simulink model "Two_Level_SVM_No_PV_No_Control_Average_Benchmark_v2"  (R2022b)
settings: Solver=FixedStepAuto  StartTime=0.0  StopTime=5  FixedStep=1e-7  RelTol=1e-3
model workspace (MAT data in the model file):
  Phase_Shift = Simulink.Parameter
  Phase_Shift.Value = 0.1974
  Phase_Shift.DataType = 'auto'
  Phase_Shift.Complexity = 'real'
  Phase_Shift.Dimensions = [1 1]
  Vrms_p = Simulink.Parameter
  Vrms_p.Value = 285.7229
  Vrms_p.DataType = 'auto'
  Vrms_p.Complexity = 'real'
  Vrms_p.Dimensions = [1 1]
libraries: slpidlib x5, spsThreePhaseSeriesRLCBranchLib x4, spsThreePhaseVIMeasurementLib x4, spsControlledCurrentSourceLib x3, spsControlledVoltageSourceLib x3, spsGroundLib x2, spsabctodq0Lib x2, spsdq0toabcLib x1, spsDCVoltageSourceLib x1, spsThreePhaseProgrammableVoltageSourceLib x1, eeGeneralControl x1, spsabctoAlphaBetaZeroLib x1
settings Model: Creator=Jacob  LastModifiedBy=buckb
settings ModelReferenceCC: EnableRefExpFcnMdlSchedulingChecks=on

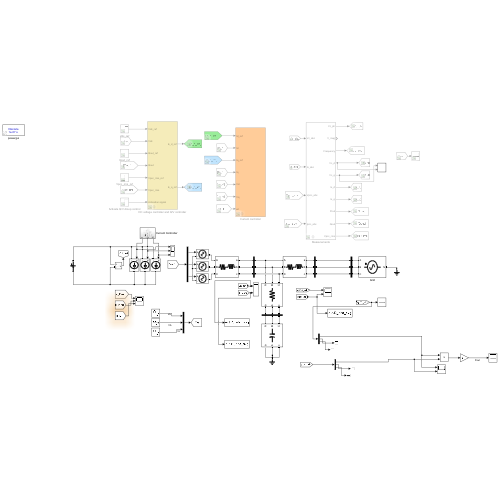
[thumbnail: Simulink's stored preview of the top-level diagram]
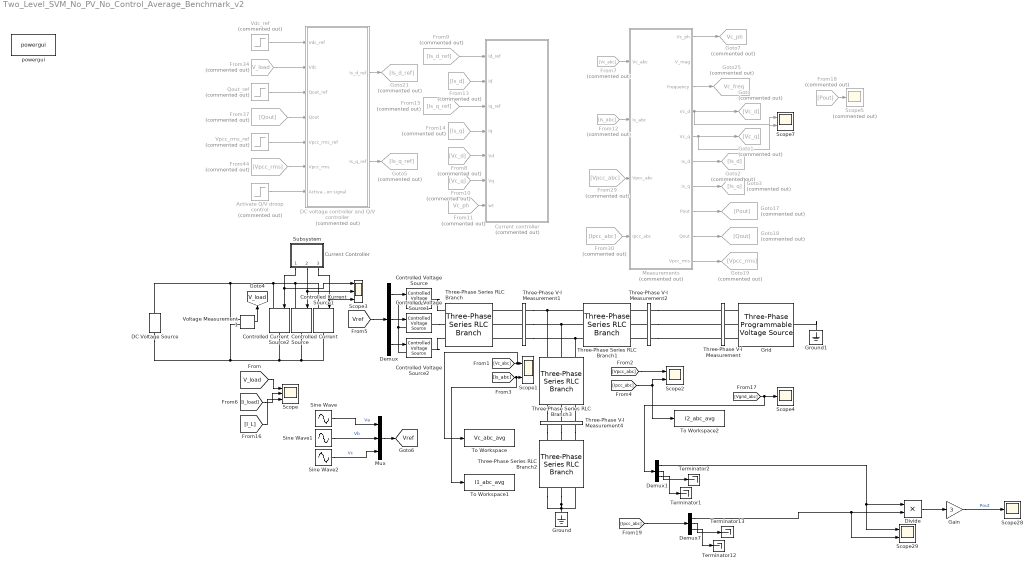
== system Two_Level_SVM_No_PV_No_Control_Average_Benchmark_v2 ==
  note: Current Controller
  Activate Q/V droop control : Step  Commented=on  Time=3  After=0  SampleTime=0
  Controlled Current Source : spsControlledCurrentSourceLib/Controlled Current Source  Initialize=on  Source_Type=AC  Amplitude=0  Phase=0  Frequency=0  Measurements=None
  Controlled Current Source1 : spsControlledCurrentSourceLib/Controlled Current Source  Initialize=on  Source_Type=AC  Amplitude=0  Phase=0  Frequency=0  Measurements=None
  Controlled Current Source2 : spsControlledCurrentSourceLib/Controlled Current Source  Initialize=on  Source_Type=AC  Amplitude=0  Phase=0  Frequency=0  Measurements=None
  Controlled Voltage Source : spsControlledVoltageSourceLib/Controlled Voltage Source  Initialize=on  Source_Type=AC  Amplitude=0  Phase=0  Frequency=0  Measurements=None
  Controlled Voltage Source1 : spsControlledVoltageSourceLib/Controlled Voltage Source  Initialize=on  Source_Type=AC  Amplitude=0  Phase=0  Frequency=0  Measurements=None
  Controlled Voltage Source2 : spsControlledVoltageSourceLib/Controlled Voltage Source  Initialize=on  Source_Type=AC  Amplitude=0  Phase=0  Frequency=0  Measurements=None
  Current controller : Subsystem  Commented=on  mask{Kp_current_loop=0.59, Ki_current_loop=30, L1=3e-03}
      mask prompts: Kp_current_loop "Proportional parameter of current loop"; Ki_current_loop "Integral parameter of current loop"; L1 "Inverter-side inductor value [H]"
      mask TypeOptions Kp_current_loop: Discrete PID Controller/P | Discrete PID Controller1/P
      mask TypeOptions Ki_current_loop: Discrete PID Controller/I | Discrete PID Controller1/I
      mask TypeOptions L1: L/Gain | L1/Gain
  DC Voltage Source : spsDCVoltageSourceLib/DC Voltage Source  Amplitude=1000  Measurements=None
  DC voltage controller and Q/V controller : Subsystem  Commented=on  mask(DC voltage controller and Q/V controller){Kp_vdc_control=0.05, Ki_vdc_control=10, Kp_QV_control=1e-3, Ki_QV_control=1e-2, Dq=4.1667e+03}
      mask prompts: Kp_vdc_control "Proportional parameter of DC voltage controller"; Ki_vdc_control "Integral parameter of DC voltage controller"; Kp_QV_control "Proportional parameter of Q/V controller"; Ki_QV_control "Integral parameter of Q/V controller"; Dq "Q/V droop constant [Var/V]"
      mask TypeOptions Kp_vdc_control: Discrete PID Controller/P
      mask TypeOptions Ki_vdc_control: Discrete PID Controller/I
      mask TypeOptions Kp_QV_control: Discrete PID Controller3/P
      mask TypeOptions Ki_QV_control: Discrete PID Controller3/I
      mask TypeOptions Dq: Dq/Gain
      mask DialogControl ParameterGroupVar1 Prompt: DC voltage controller
      mask DialogControl ParameterGroupVar2 Prompt: Q/V controller
  Demux : Demux  Outputs=3
  Demux1 : Demux  Outputs=3
  Demux7 : Demux  Outputs=3
  Divide : Product  Inputs=**
  From10 : From  Commented=on  GotoTag=Vc_q
  From11 : From  Commented=on  GotoTag=Vc_ph  TagVisibility=global
  From12 : From  Commented=on  GotoTag=Is_abc  TagVisibility=global
  From13 : From  Commented=on  GotoTag=Is_d
  From14 : From  Commented=on  GotoTag=Is_q
  From15 : From  Commented=on  GotoTag=Is_q_ref
  From18 : From  Commented=on  GotoTag=Pout
  From29 : From  Commented=on  GotoTag=Vpcc_abc  TagVisibility=global
  From30 : From  Commented=on  GotoTag=Ipcc_abc  TagVisibility=global
  From34 : From  Commented=on  GotoTag=V_load  TagVisibility=global
  From37 : From  Commented=on  GotoTag=Qout
  From44 : From  Commented=on  GotoTag=Vpcc_rms
  From7 : From  Commented=on  GotoTag=Vc_abc  TagVisibility=global
  From8 : From  Commented=on  GotoTag=Vc_d
  From9 : From  Commented=on  GotoTag=Is_d_ref
  Gain : Gain  Gain=3
  Goto : Goto  Commented=on  GotoTag=Vc_d
  Goto1 : Goto  Commented=on  GotoTag=Vc_q
  Goto17 : Goto  Commented=on  GotoTag=Pout
  Goto18 : Goto  Commented=on  GotoTag=Qout
  Goto19 : Goto  Commented=on  GotoTag=Vpcc_rms
  Goto2 : Goto  Commented=on  GotoTag=Is_d
  Goto21 : Goto  Commented=on  GotoTag=Is_d_ref
  Goto25 : Goto  Commented=on  GotoTag=Vc_freq  TagVisibility=global
  Goto3 : Goto  Commented=on  GotoTag=Is_q
  Goto5 : Goto  Commented=on  GotoTag=Is_q_ref
  Goto7 : Goto  Commented=on  GotoTag=Vc_ph  TagVisibility=global
  Grid : spsThreePhaseProgrammableVoltageSourceLib/Three-Phase Programmable Voltage Source  PositiveSequence="[480  0 60]"  VariationEntity=None  VariationType=Table of time-amplitude pairs  VariationTypeAlt=Step  VariationStep=-0.1  VariationRate=10  VariationMagnitude=0.3  VariationFrequency=2  VariationTiming=[5.5 6.5]  VariationPhaseA=off  Amplitudes=[1 0.96 1.02]  TimeValues=[0 7 8.5]  HarmonicGeneration=off  HarmonicA=[3 0.2 -25 0]  HarmonicB=[2 0.15 35 2]  Timing="[0.05  3]"  BusType=swing  Pref=0  Qref=0  Qmin=-inf  Qmax=inf
  Ground : spsGroundLib/Ground  LConnTagsString=a
  Ground1 : spsGroundLib/Ground  LConnTagsString=a
  Measurements : Subsystem  Commented=on  mask{Kp_PLL=100, Ki_PLL=1e5}
      mask prompts: Kp_PLL "Proportional parameter of PLL"; Ki_PLL "Integral parameter of PLL"
      mask TypeOptions Kp_PLL: Phase Locked Loop (PLL)/Discrete PID Controller/P
      mask TypeOptions Ki_PLL: Phase Locked Loop (PLL)/Discrete PID Controller/I
  Mux : Mux  Inputs=3
  Qout_ref : Step  Commented=on  Time=0  After=0  SampleTime=0
  Scope : Scope  NumInputPorts=3
  Scope{1..2,7,29} (4 alike) : Scope  NumInputPorts=2
  Scope28 : Scope
  Scope3 : Scope  NumInputPorts=3
  Scope4 : Scope
  Scope5 : Scope  Commented=on
  Sine Wave : Sin  Amplitude=Vrms_p*sqrt(2)  Frequency=2*pi*60  Phase=Phase_Shift  SampleTime=0
  Sine Wave1 : Sin  Amplitude=Vrms_p*sqrt(2)  Frequency=2*pi*60  Phase=4*pi/3+Phase_Shift  SampleTime=0
  Sine Wave2 : Sin  Amplitude=Vrms_p*sqrt(2)  Frequency=2*pi*60  Phase=2*pi/3+Phase_Shift  SampleTime=0
  Subsystem : Subsystem
  Terminator{1..2,12..13} (4 alike) : Terminator
  Three-Phase Series RLC Branch : spsThreePhaseSeriesRLCBranchLib/Three-Phase Series RLC Branch  LConnTagsString=A|B|C  RConnTagsString=A|B|C  BranchType=RL  Resistance=0.03  Inductance=3e-04  Capacitance=1e-6  Measurements=None
  Three-Phase Series RLC Branch1 : spsThreePhaseSeriesRLCBranchLib/Three-Phase Series RLC Branch  LConnTagsString=A|B|C  RConnTagsString=A|B|C  BranchType=RL  Resistance=0.0053  Inductance=9.3183e-04  Capacitance=1e-6  Measurements=None
  Three-Phase Series RLC Branch2 : spsThreePhaseSeriesRLCBranchLib/Three-Phase Series RLC Branch  LConnTagsString=A|B|C  RConnTagsString=A|B|C  BranchType=C  Resistance=1  Inductance=1e-3  Capacitance=9.7860e-5  Measurements=None
  Three-Phase Series RLC Branch3 : spsThreePhaseSeriesRLCBranchLib/Three-Phase Series RLC Branch  LConnTagsString=A|B|C  RConnTagsString=A|B|C  BranchType=R  Resistance=1  Inductance=1e-3  Capacitance=9.7860e-5  Measurements=None
  Three-Phase V-I Measurement : spsThreePhaseVIMeasurementLib/Three-Phase V-I Measurement  VoltageMeasurement=phase-to-ground  SetLabelV=on  LabelV=Vgrid_abc  Vpu=off  VpuLL=off  CurrentMeasurement=yes  SetLabelI=on  LabelI=Igrid_abc  Ipu=off  Pbase=100e6  Vbase=500e3  OutputType=Complex  PhasorSimulation=off  PSBequivalent=0
  Three-Phase V-I Measurement1 : spsThreePhaseVIMeasurementLib/Three-Phase V-I Measurement  VoltageMeasurement=phase-to-ground  SetLabelV=on  LabelV=Vrc_abc  Vpu=off  VpuLL=off  CurrentMeasurement=yes  SetLabelI=on  LabelI=Is_abc  Ipu=off  Pbase=100e6  Vbase=500e3  OutputType=Complex  PhasorSimulation=off  PSBequivalent=0
  Three-Phase V-I Measurement2 : spsThreePhaseVIMeasurementLib/Three-Phase V-I Measurement  VoltageMeasurement=phase-to-ground  SetLabelV=on  LabelV=Vpcc_abc  Vpu=off  VpuLL=off  CurrentMeasurement=yes  SetLabelI=on  LabelI=Ipcc_abc  Ipu=off  Pbase=100e6  Vbase=500e3  OutputType=Complex  PhasorSimulation=off  PSBequivalent=0
  Three-Phase V-I Measurement4 : spsThreePhaseVIMeasurementLib/Three-Phase V-I Measurement  VoltageMeasurement=phase-to-ground  SetLabelV=on  LabelV=Vc_abc  Vpu=off  VpuLL=off  CurrentMeasurement=yes  SetLabelI=on  LabelI=Ic_abc  Ipu=off  Pbase=100e6  Vbase=500e3  OutputType=Complex  PhasorSimulation=off  PSBequivalent=0
  To Workspace : ToWorkspace  VariableName=Vc_abc_avg  SaveFormat=Timeseries  SampleTime=-1
  To Workspace1 : ToWorkspace  VariableName=I1_abc_avg  SaveFormat=Timeseries  SampleTime=-1
  To Workspace2 : ToWorkspace  VariableName=I2_abc_avg  SaveFormat=Timeseries  SampleTime=-1
  Vdc_ref : Step  Commented=on  Time=0.5  Before=1000  After=1000  SampleTime=0
  Voltage Measurement1 : spsVoltageMeasurementLib/Voltage Measurement  PhasorSimulation=off  OutputType=Complex  PSBequivalent=0
  Vpcc_rms_ref : Step  Commented=on  Time=0.5  Before=480  After=480  SampleTime=0
  powergui : spspowerguiLib/powergui  Priority=1  SimulationMode=Discrete  SampleTime=1e-7  frequency=60  Iterations=50  frequencyindice=0  Pbase=100e6  ErrMax=1e-4  UnitsV=kV  UnitsW=MW  buscounter=0  FunctionMessages=off  echomessages=off  EnableUseOfTLC=off  CurrentSourceSwitches=off  DisableSnubberDevices=off  DisableRonSwitches=off  DisableVfSwitches=off  DisplayEquations=off  AutomaticDiscreteSolvers=off  SolverType=Tustin/Backward Euler (TBE)  Interpol=off  ExternalGateDelay=off  methode=off  Ts=100  x0status=blocks  SPID=on  SwTol=0  HookPort=off  NonlinearTolerance=1e-4  nMaxIteration=100  ContinueOnMaxIteration=off  RestoreLinks=warning  ResistiveCurrentMeasurement=off  Frange=[0:2:500]  Ylog=off  Xlog=on  ShowGrid=off  save=off  variable=ZData  structure=0  ZoomFFT=off  StartTime=0.0  cycles=1  DisplayStyle=1  fundamental=60  FreqAxis=off  MaxFrequency=1000  frequencyindicesteady=1  RmsSteady=1  display=off
  tag scope: V_load=global, Vref=global
  wires:
  Voltage Measurement1/1 -> [V_load]
  [V_load] -> Scope/1
  [Vpcc_abc] -> Scope2/1
  [Ipcc_abc] -> To Workspace2/1, Scope2/2
  Subsystem/1(Out1) -> Controlled Current Source2/1, Scope3/1
  Subsystem/2(Out2) -> Controlled Current Source/1, Scope3/2
  Subsystem/3(Out3) -> Controlled Current Source1/1, Scope3/3
  Demux/1 -> Controlled Voltage Source/1
  Demux/2 -> Controlled Voltage Source1/1
  Demux/3 -> Controlled Voltage Source2/1
  From8/1 -> Current controller/5(Vd)
  From10/1 -> Current controller/6(Vq)
  From11/1 -> Current controller/7(wt)
  From14/1 -> Current controller/4(Iq)
  From13/1 -> Current controller/2(Id)
  From7/1 -> Measurements/1(Vc_abc)
  From12/1 -> Measurements/2(Is_abc)
  Measurements/4(Vc_d) -> Scope7/1, Goto/1
  Measurements/5(Vc_q) -> Scope7/2, Goto1/1
  Measurements/6(Is_d) -> Goto2/1
  Measurements/7(Is_q) -> Goto3/1
  Qout_ref/1 -> DC voltage controller and Q/V controller/3(Qout_ref)
  From44/1 -> DC voltage controller and Q/V controller/6(Vpcc_rms)
  DC voltage controller and Q/V controller/2(Is_q_ref) -> Goto5/1
  Activate Q/V droop control/1 -> DC voltage controller and Q/V controller/7(Activation signal)
  Vpcc_rms_ref/1 -> DC voltage controller and Q/V controller/5(Vpcc_rms_ref)
  From37/1 -> DC voltage controller and Q/V controller/4(Qout)
  DC voltage controller and Q/V controller/1(Is_d_ref) -> Goto21/1
  Vdc_ref/1 -> DC voltage controller and Q/V controller/1(Vdc_ref)
  From29/1 -> Measurements/3(Vpcc_abc)
  From30/1 -> Measurements/4(Ipcc_abc)
  Measurements/8(Pout) -> Goto17/1
  Measurements/9(Qout) -> Goto18/1
  Measurements/10(Vpcc_rms) -> Goto19/1
  Measurements/3(Frequency) -> Goto25/1
  From15/1 -> Current controller/3(Iq_ref)
  From9/1 -> Current controller/1(Id_ref)
  Measurements/1(Vc_ph) -> Goto7/1
  From18/1 -> Scope5/1
  [I_L] -> Scope/3
  [I_load] -> Scope/2
  From34/1 -> DC voltage controller and Q/V controller/2(Vdc)
  [Is_abc] -> To Workspace1/1, Scope1/2
  [Vc_abc] -> To Workspace/1, Scope1/1
  Sine Wave1/1 -> Mux/2  "Vb"
  Sine Wave/1 -> Mux/1  "Va"
  Sine Wave2/1 -> Mux/3  "Vc"
  Mux/1 -> [Vref]
  [Vref] -> Demux/1
  Demux7/2 -> Terminator13/1
  Demux7/1 -> Scope29/2, Divide/2
  Demux1/1 -> Scope29/1, Divide/1
  Demux7/3 -> Terminator12/1
  [Ipcc_abc] -> Demux7/1
  Gain/1 -> Scope28/1  "Pout"
  Divide/1 -> Gain/1
  Demux1/3 -> Terminator1/1
  Demux1/2 -> Terminator2/1
  [Vgrid_abc] -> Demux1/1, Scope4/1
  connections:
  DC Voltage Source/RConn1 -- Voltage Measurement1/LConn1 -- Controlled Current Source2/LConn1 -- Controlled Current Source1/LConn1 -- Controlled Current Source/LConn1
  Three-Phase V-I Measurement1/RConn3 -- Three-Phase Series RLC Branch3/LConn3 -- Three-Phase Series RLC Branch1/LConn3
  Three-Phase V-I Measurement1/RConn1 -- Three-Phase Series RLC Branch3/LConn1 -- Three-Phase Series RLC Branch1/LConn1
  Three-Phase V-I Measurement1/RConn2 -- Three-Phase Series RLC Branch3/LConn2 -- Three-Phase Series RLC Branch1/LConn2
  Three-Phase V-I Measurement1/LConn3 -- Three-Phase Series RLC Branch/RConn3
  Three-Phase V-I Measurement2/RConn3 -- Three-Phase V-I Measurement/LConn3
  Three-Phase V-I Measurement2/RConn1 -- Three-Phase V-I Measurement/LConn1
  Grid/RConn1 -- Three-Phase V-I Measurement/RConn1
  Grid/RConn2 -- Three-Phase V-I Measurement/RConn2
  Ground1/LConn1 -- Grid/LConn1
  Three-Phase V-I Measurement1/LConn1 -- Three-Phase Series RLC Branch/RConn1
  Grid/RConn3 -- Three-Phase V-I Measurement/RConn3
  Three-Phase V-I Measurement1/LConn2 -- Three-Phase Series RLC Branch/RConn2
  Three-Phase V-I Measurement2/RConn2 -- Three-Phase V-I Measurement/LConn2
  Controlled Voltage Source/LConn1 -- Controlled Voltage Source2/LConn1 -- Controlled Voltage Source1/LConn1
  Controlled Voltage Source/RConn1 -- Three-Phase Series RLC Branch/LConn1
  Controlled Voltage Source1/RConn1 -- Three-Phase Series RLC Branch/LConn2
  Controlled Voltage Source2/RConn1 -- Three-Phase Series RLC Branch/LConn3
  Three-Phase V-I Measurement2/LConn1 -- Three-Phase Series RLC Branch1/RConn1
  Three-Phase V-I Measurement2/LConn2 -- Three-Phase Series RLC Branch1/RConn2
  Three-Phase V-I Measurement2/LConn3 -- Three-Phase Series RLC Branch1/RConn3
  Controlled Current Source/RConn1 -- Controlled Current Source1/RConn1 -- Controlled Current Source2/RConn1 -- DC Voltage Source/LConn1 -- Voltage Measurement1/LConn2
  Ground/LConn1 -- Three-Phase Series RLC Branch2/RConn1 -- Three-Phase Series RLC Branch2/RConn3 -- Three-Phase Series RLC Branch2/RConn2
  Three-Phase V-I Measurement4/LConn3 -- Three-Phase Series RLC Branch3/RConn3
  Three-Phase Series RLC Branch3/RConn2 -- Three-Phase V-I Measurement4/LConn2
  Three-Phase Series RLC Branch3/RConn1 -- Three-Phase V-I Measurement4/LConn1
  Three-Phase V-I Measurement4/RConn1 -- Three-Phase Series RLC Branch2/LConn1
  Three-Phase V-I Measurement4/RConn2 -- Three-Phase Series RLC Branch2/LConn2
  Three-Phase V-I Measurement4/RConn3 -- Three-Phase Series RLC Branch2/LConn3

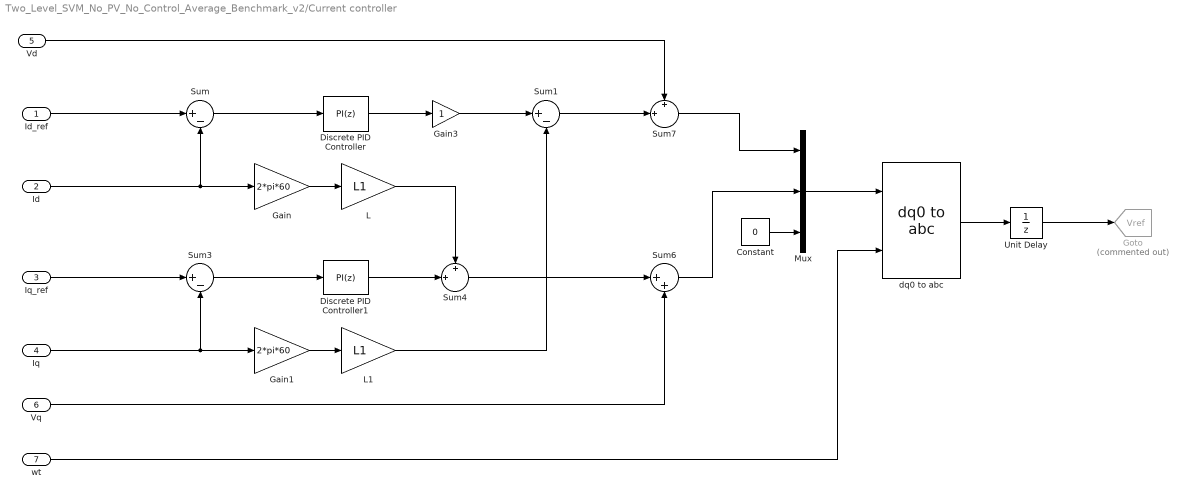
== system Two_Level_SVM_No_PV_No_Control_Average_Benchmark_v2/Current controller ==
  Id_ref : Inport
  Id : Inport  Port=2
  Iq_ref : Inport  Port=3
  Iq : Inport  Port=4
  Vd : Inport  Port=5
  Vq : Inport  Port=6
  wt : Inport  Port=7
  Constant : Constant  Value=0
  Discrete PID Controller : slpidlib/PID Controller  Controller=PI  Form=Parallel  TimeDomain=Discrete-time  UseExternalTs=off  SampleTime=-1  IntegratorMethod=Forward Euler  FilterMethod=Forward Euler  ControllerParametersSource=internal  P=Kp_current_loop  I=Ki_current_loop  UseKiTs=off  D=0  N=100  UseFilter=on  TunerSelectOption=Transfer Function Based (PID Tuner App)  InitialConditionSource=internal  InitialConditionForIntegrator=0  InitialConditionForFilter=0  DifferentiatorICPrevScaledInput=0  ExternalReset=none  TrackingMode=off  Kt=1  LimitOutput=off  SatLimitsSource=internal  UpperSaturationLimit=inf  LowerSaturationLimit=-inf  LinearizeAsGain=off  AntiWindupMode=none  Kb=1  LimitIntegrator=off  UpperIntegratorSaturationLimit=inf  LowerIntegratorSaturationLimit=-inf  POutMin=[]  POutMax=[]  IOutMin=[]  IOutMax=[]  DOutMin=[]  DOutMax=[]  NOutMin=[]  NOutMax=[]  SumOutMin=[]  SumOutMax=[]  SaturationOutMin=[]  SaturationOutMax=[]  PParamMin=[]  PParamMax=[]  IParamMin=[]  IParamMax=[]  DParamMin=[]  DParamMax=[]  NParamMin=[]  NParamMax=[]  KbParamMin=[]  KbParamMax=[]  KtParamMin=[]  KtParamMax=[]  KbOutMin=[]  KbOutMax=[]  KtOutMin=[]  KtOutMax=[]  IntegratorOutMin=[]  IntegratorOutMax=[]  FilterOutMin=[]  FilterOutMax=[]  SumI1OutMin=[]  SumI1OutMax=[]  SumI2OutMin=[]  SumI2OutMax=[]  SumI3OutMin=[]  SumI3OutMax=[]  SumI4OutMin=[]  SumI4OutMax=[]  SumDOutMin=[]  SumDOutMax=[]  DifferentiatorOutMin=[]  DifferentiatorOutMax=[]  FilterDiffOutCoefMin=[]  FilterDiffOutCoefMax=[]  ReciprocalOutMin=[]  ReciprocalOutMax=[]  SumDenOutMin=[]  SumDenOutMax=[]  SumNumOutMin=[]  SumNumOutMax=[]  DivideOutMin=[]  DivideOutMax=[]  UdiffTsProdOutMin=[]  UdiffTsProdOutMax=[]  NTsProdOutMin=[]  NTsProdOutMax=[]  UintegralTsProdOutMin=[]  UintegralTsProdOutMax=[]  UngainTsProdOutMin=[]  UngainTsProdOutMax=[]  ClampingZeroOutDataTypeStr=Inherit: Inherit via back propagation  ClampingZeroOutMin=[]  ClampingZeroOutMax=[]  FilterDenConstantOutDataTypeStr=Inherit: Inherit via back propagation  FilterDenConstantOutMin=[]  FilterDenConstantOutMax=[]  PCopyOutDataTypeStr=Inherit: Inherit via back propagation  PCopyOutMin=[]  PCopyOutMax=[]  NCopyOutDataTypeStr=Inherit: Inherit via back propagation  NCopyOutMin=[]  NCopyOutMax=[]  IntegratorContinuousStateAttributes=''  IntegratorStateMustResolveToSignalObject=off  IntegratorRTWStateStorageClass=Auto  FilterContinuousStateAttributes=''  FilterStateMustResolveToSignalObject=off  FilterRTWStateStorageClass=Auto  ParallelPVariant=InternalParameters  IdealPVariant=Disabled  IVariant=InternalParameters  DVariant=Disabled  IntegratorVariant=Discrete  SatVariant=Disabled  AWVariant=Passthrough  PCopyVariant=Disabled  TRVariant=Disabled  FdbkBlocksVariant=Forward  IdealPFdbkVariant=Disabled  SatFdbkVariant=Disabled  DerivativeFilterVariant=Disabled  NVariant=Disabled  NCopyVariant=Disabled_SignalSpec  FilterICVariant=Disabled  IntegratorICVariant=InternalICs  ExternalResetVariant=Disabled  TRSumVariant=Passthrough  SumFdbkVariant=Disabled  SumVariant=Sum_PI  TsampFilterVariant=InternalTs  TsampNgainVariant=Passthrough  TsampIntegralVariant=Passthrough  ExternalSaturationOutDataTypeStr=Inherit: Same as second input
  Discrete PID Controller1 : slpidlib/PID Controller  Controller=PI  Form=Parallel  TimeDomain=Discrete-time  UseExternalTs=off  SampleTime=-1  IntegratorMethod=Forward Euler  FilterMethod=Forward Euler  ControllerParametersSource=internal  P=Kp_current_loop  I=Ki_current_loop  UseKiTs=off  D=0  N=100  UseFilter=on  TunerSelectOption=Transfer Function Based (PID Tuner App)  InitialConditionSource=internal  InitialConditionForIntegrator=0  InitialConditionForFilter=0  DifferentiatorICPrevScaledInput=0  ExternalReset=none  TrackingMode=off  Kt=1  LimitOutput=off  SatLimitsSource=internal  UpperSaturationLimit=inf  LowerSaturationLimit=-inf  LinearizeAsGain=off  AntiWindupMode=none  Kb=1  LimitIntegrator=off  UpperIntegratorSaturationLimit=inf  LowerIntegratorSaturationLimit=-inf  POutMin=[]  POutMax=[]  IOutMin=[]  IOutMax=[]  DOutMin=[]  DOutMax=[]  NOutMin=[]  NOutMax=[]  SumOutMin=[]  SumOutMax=[]  SaturationOutMin=[]  SaturationOutMax=[]  PParamMin=[]  PParamMax=[]  IParamMin=[]  IParamMax=[]  DParamMin=[]  DParamMax=[]  NParamMin=[]  NParamMax=[]  KbParamMin=[]  KbParamMax=[]  KtParamMin=[]  KtParamMax=[]  KbOutMin=[]  KbOutMax=[]  KtOutMin=[]  KtOutMax=[]  IntegratorOutMin=[]  IntegratorOutMax=[]  FilterOutMin=[]  FilterOutMax=[]  SumI1OutMin=[]  SumI1OutMax=[]  SumI2OutMin=[]  SumI2OutMax=[]  SumI3OutMin=[]  SumI3OutMax=[]  SumI4OutMin=[]  SumI4OutMax=[]  SumDOutMin=[]  SumDOutMax=[]  DifferentiatorOutMin=[]  DifferentiatorOutMax=[]  FilterDiffOutCoefMin=[]  FilterDiffOutCoefMax=[]  ReciprocalOutMin=[]  ReciprocalOutMax=[]  SumDenOutMin=[]  SumDenOutMax=[]  SumNumOutMin=[]  SumNumOutMax=[]  DivideOutMin=[]  DivideOutMax=[]  UdiffTsProdOutMin=[]  UdiffTsProdOutMax=[]  NTsProdOutMin=[]  NTsProdOutMax=[]  UintegralTsProdOutMin=[]  UintegralTsProdOutMax=[]  UngainTsProdOutMin=[]  UngainTsProdOutMax=[]  ClampingZeroOutDataTypeStr=Inherit: Inherit via back propagation  ClampingZeroOutMin=[]  ClampingZeroOutMax=[]  FilterDenConstantOutDataTypeStr=Inherit: Inherit via back propagation  FilterDenConstantOutMin=[]  FilterDenConstantOutMax=[]  PCopyOutDataTypeStr=Inherit: Inherit via back propagation  PCopyOutMin=[]  PCopyOutMax=[]  NCopyOutDataTypeStr=Inherit: Inherit via back propagation  NCopyOutMin=[]  NCopyOutMax=[]  IntegratorContinuousStateAttributes=''  IntegratorStateMustResolveToSignalObject=off  IntegratorRTWStateStorageClass=Auto  FilterContinuousStateAttributes=''  FilterStateMustResolveToSignalObject=off  FilterRTWStateStorageClass=Auto  ParallelPVariant=InternalParameters  IdealPVariant=Disabled  IVariant=InternalParameters  DVariant=Disabled  IntegratorVariant=Discrete  SatVariant=Disabled  AWVariant=Passthrough  PCopyVariant=Disabled  TRVariant=Disabled  FdbkBlocksVariant=Forward  IdealPFdbkVariant=Disabled  SatFdbkVariant=Disabled  DerivativeFilterVariant=Disabled  NVariant=Disabled  NCopyVariant=Disabled_SignalSpec  FilterICVariant=Disabled  IntegratorICVariant=InternalICs  ExternalResetVariant=Disabled  TRSumVariant=Passthrough  SumFdbkVariant=Disabled  SumVariant=Sum_PI  TsampFilterVariant=InternalTs  TsampNgainVariant=Passthrough  TsampIntegralVariant=Passthrough  ExternalSaturationOutDataTypeStr=Inherit: Same as second input
  Gain : Gain  Gain=2*pi*60
  Gain1 : Gain  Gain=2*pi*60
  Gain3 : Gain
  Goto : Goto  Commented=on  GotoTag=Vref  TagVisibility=global
  L : Gain  Gain=L1
  L1 : Gain  Gain=L1
  Mux : Mux  Inputs=3
  Sum : Sum  Inputs=|+-
  Sum1 : Sum  Inputs=|+-
  Sum3 : Sum  Inputs=|+-
  Sum4 : Sum  Inputs=+|+||
  Sum6 : Sum  Inputs=|++
  Sum7 : Sum  Inputs=+|+||
  Unit Delay : UnitDelay  SampleTime=-1  HasFrameUpgradeWarning=on
  dq0 to abc : spsdq0toabcLib/dq0 to abc  Alignment=Aligned with phase A axis
  wires:
  Iq/1 -> Gain1/1, Sum3/2
  Constant/1 -> Mux/3
  wt/1 -> dq0 to abc/2
  Sum4/1 -> Sum6/1
  Id/1 -> Gain/1, Sum/2
  Vd/1 -> Sum7/1
  Mux/1 -> dq0 to abc/1
  Sum1/1 -> Sum7/2
  Gain/1 -> L/1
  Discrete PID Controller/1 -> Gain3/1
  Sum/1 -> Discrete PID Controller/1
  Sum3/1 -> Discrete PID Controller1/1
  Vq/1 -> Sum6/2
  Gain1/1 -> L1/1
  L/1 -> Sum4/1
  Sum7/1 -> Mux/1
  L1/1 -> Sum1/2
  Sum6/1 -> Mux/2
  Iq_ref/1 -> Sum3/1
  Id_ref/1 -> Sum/1
  Gain3/1 -> Sum1/1
  Discrete PID Controller1/1 -> Sum4/2
  dq0 to abc/1 -> Unit Delay/1
  Unit Delay/1 -> Goto/1

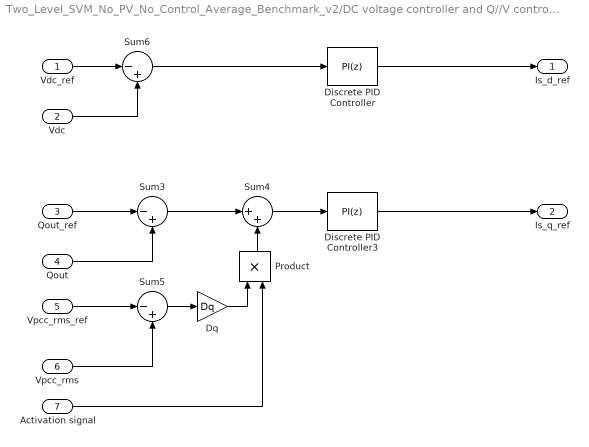
== system Two_Level_SVM_No_PV_No_Control_Average_Benchmark_v2/DC voltage controller and Q//V controller ==
  Vdc_ref : Inport
  Vdc : Inport  Port=2
  Qout_ref : Inport  Port=3
  Qout : Inport  Port=4
  Vpcc_rms_ref : Inport  Port=5
  Vpcc_rms : Inport  Port=6
  Activation signal : Inport  Port=7
  Discrete PID Controller : slpidlib/PID Controller  Controller=PI  Form=Parallel  TimeDomain=Discrete-time  UseExternalTs=off  SampleTime=-1  IntegratorMethod=Forward Euler  FilterMethod=Forward Euler  ControllerParametersSource=internal  P=Kp_vdc_control  I=Ki_vdc_control  UseKiTs=off  D=0  N=100  UseFilter=on  TunerSelectOption=Transfer Function Based (PID Tuner App)  InitialConditionSource=internal  InitialConditionForIntegrator=0  InitialConditionForFilter=0  DifferentiatorICPrevScaledInput=0  ExternalReset=none  TrackingMode=off  Kt=1  LimitOutput=off  SatLimitsSource=internal  UpperSaturationLimit=inf  LowerSaturationLimit=-inf  LinearizeAsGain=off  AntiWindupMode=none  Kb=1  LimitIntegrator=off  UpperIntegratorSaturationLimit=inf  LowerIntegratorSaturationLimit=-inf  POutMin=[]  POutMax=[]  IOutMin=[]  IOutMax=[]  DOutMin=[]  DOutMax=[]  NOutMin=[]  NOutMax=[]  SumOutMin=[]  SumOutMax=[]  SaturationOutMin=[]  SaturationOutMax=[]  PParamMin=[]  PParamMax=[]  IParamMin=[]  IParamMax=[]  DParamMin=[]  DParamMax=[]  NParamMin=[]  NParamMax=[]  KbParamMin=[]  KbParamMax=[]  KtParamMin=[]  KtParamMax=[]  KbOutMin=[]  KbOutMax=[]  KtOutMin=[]  KtOutMax=[]  IntegratorOutMin=[]  IntegratorOutMax=[]  FilterOutMin=[]  FilterOutMax=[]  SumI1OutMin=[]  SumI1OutMax=[]  SumI2OutMin=[]  SumI2OutMax=[]  SumI3OutMin=[]  SumI3OutMax=[]  SumI4OutMin=[]  SumI4OutMax=[]  SumDOutMin=[]  SumDOutMax=[]  DifferentiatorOutMin=[]  DifferentiatorOutMax=[]  FilterDiffOutCoefMin=[]  FilterDiffOutCoefMax=[]  ReciprocalOutMin=[]  ReciprocalOutMax=[]  SumDenOutMin=[]  SumDenOutMax=[]  SumNumOutMin=[]  SumNumOutMax=[]  DivideOutMin=[]  DivideOutMax=[]  UdiffTsProdOutMin=[]  UdiffTsProdOutMax=[]  NTsProdOutMin=[]  NTsProdOutMax=[]  UintegralTsProdOutMin=[]  UintegralTsProdOutMax=[]  UngainTsProdOutMin=[]  UngainTsProdOutMax=[]  ClampingZeroOutDataTypeStr=Inherit: Inherit via back propagation  ClampingZeroOutMin=[]  ClampingZeroOutMax=[]  FilterDenConstantOutDataTypeStr=Inherit: Inherit via back propagation  FilterDenConstantOutMin=[]  FilterDenConstantOutMax=[]  PCopyOutDataTypeStr=Inherit: Inherit via back propagation  PCopyOutMin=[]  PCopyOutMax=[]  NCopyOutDataTypeStr=Inherit: Inherit via back propagation  NCopyOutMin=[]  NCopyOutMax=[]  IntegratorContinuousStateAttributes=''  IntegratorStateMustResolveToSignalObject=off  IntegratorRTWStateStorageClass=Auto  FilterContinuousStateAttributes=''  FilterStateMustResolveToSignalObject=off  FilterRTWStateStorageClass=Auto  ParallelPVariant=InternalParameters  IdealPVariant=Disabled  IVariant=InternalParameters  DVariant=Disabled  IntegratorVariant=Discrete  SatVariant=Disabled  AWVariant=Passthrough  PCopyVariant=Disabled  TRVariant=Disabled  FdbkBlocksVariant=Forward  IdealPFdbkVariant=Disabled  SatFdbkVariant=Disabled  DerivativeFilterVariant=Disabled  NVariant=Disabled  NCopyVariant=Disabled_SignalSpec  FilterICVariant=Disabled  IntegratorICVariant=InternalICs  ExternalResetVariant=Disabled  TRSumVariant=Passthrough  SumFdbkVariant=Disabled  SumVariant=Sum_PI  TsampFilterVariant=InternalTs  TsampNgainVariant=Passthrough  TsampIntegralVariant=Passthrough  ExternalSaturationOutDataTypeStr=Inherit: Same as second input
  Discrete PID Controller3 : slpidlib/PID Controller  Controller=PI  Form=Parallel  TimeDomain=Discrete-time  UseExternalTs=off  SampleTime=-1  IntegratorMethod=Forward Euler  FilterMethod=Forward Euler  ControllerParametersSource=internal  P=Kp_QV_control  I=Ki_QV_control  UseKiTs=off  D=0  N=100  UseFilter=on  TunerSelectOption=Transfer Function Based (PID Tuner App)  InitialConditionSource=internal  InitialConditionForIntegrator=0  InitialConditionForFilter=0  DifferentiatorICPrevScaledInput=0  ExternalReset=none  TrackingMode=off  Kt=1  LimitOutput=off  SatLimitsSource=internal  UpperSaturationLimit=inf  LowerSaturationLimit=-inf  LinearizeAsGain=off  AntiWindupMode=none  Kb=1  LimitIntegrator=off  UpperIntegratorSaturationLimit=inf  LowerIntegratorSaturationLimit=-inf  POutMin=[]  POutMax=[]  IOutMin=[]  IOutMax=[]  DOutMin=[]  DOutMax=[]  NOutMin=[]  NOutMax=[]  SumOutMin=[]  SumOutMax=[]  SaturationOutMin=[]  SaturationOutMax=[]  PParamMin=[]  PParamMax=[]  IParamMin=[]  IParamMax=[]  DParamMin=[]  DParamMax=[]  NParamMin=[]  NParamMax=[]  KbParamMin=[]  KbParamMax=[]  KtParamMin=[]  KtParamMax=[]  KbOutMin=[]  KbOutMax=[]  KtOutMin=[]  KtOutMax=[]  IntegratorOutMin=[]  IntegratorOutMax=[]  FilterOutMin=[]  FilterOutMax=[]  SumI1OutMin=[]  SumI1OutMax=[]  SumI2OutMin=[]  SumI2OutMax=[]  SumI3OutMin=[]  SumI3OutMax=[]  SumI4OutMin=[]  SumI4OutMax=[]  SumDOutMin=[]  SumDOutMax=[]  DifferentiatorOutMin=[]  DifferentiatorOutMax=[]  FilterDiffOutCoefMin=[]  FilterDiffOutCoefMax=[]  ReciprocalOutMin=[]  ReciprocalOutMax=[]  SumDenOutMin=[]  SumDenOutMax=[]  SumNumOutMin=[]  SumNumOutMax=[]  DivideOutMin=[]  DivideOutMax=[]  UdiffTsProdOutMin=[]  UdiffTsProdOutMax=[]  NTsProdOutMin=[]  NTsProdOutMax=[]  UintegralTsProdOutMin=[]  UintegralTsProdOutMax=[]  UngainTsProdOutMin=[]  UngainTsProdOutMax=[]  ClampingZeroOutDataTypeStr=Inherit: Inherit via back propagation  ClampingZeroOutMin=[]  ClampingZeroOutMax=[]  FilterDenConstantOutDataTypeStr=Inherit: Inherit via back propagation  FilterDenConstantOutMin=[]  FilterDenConstantOutMax=[]  PCopyOutDataTypeStr=Inherit: Inherit via back propagation  PCopyOutMin=[]  PCopyOutMax=[]  NCopyOutDataTypeStr=Inherit: Inherit via back propagation  NCopyOutMin=[]  NCopyOutMax=[]  IntegratorContinuousStateAttributes=''  IntegratorStateMustResolveToSignalObject=off  IntegratorRTWStateStorageClass=Auto  FilterContinuousStateAttributes=''  FilterStateMustResolveToSignalObject=off  FilterRTWStateStorageClass=Auto  ParallelPVariant=InternalParameters  IdealPVariant=Disabled  IVariant=InternalParameters  DVariant=Disabled  IntegratorVariant=Discrete  SatVariant=Disabled  AWVariant=Passthrough  PCopyVariant=Disabled  TRVariant=Disabled  FdbkBlocksVariant=Forward  IdealPFdbkVariant=Disabled  SatFdbkVariant=Disabled  DerivativeFilterVariant=Disabled  NVariant=Disabled  NCopyVariant=Disabled_SignalSpec  FilterICVariant=Disabled  IntegratorICVariant=InternalICs  ExternalResetVariant=Disabled  TRSumVariant=Passthrough  SumFdbkVariant=Disabled  SumVariant=Sum_PI  TsampFilterVariant=InternalTs  TsampNgainVariant=Passthrough  TsampIntegralVariant=Passthrough  ExternalSaturationOutDataTypeStr=Inherit: Same as second input
  Dq : Gain  Gain=Dq
  Product : Product
  Sum3 : Sum  Inputs=|-+
  Sum4 : Sum  Inputs=|++
  Sum5 : Sum  Inputs=|-+
  Sum6 : Sum  Inputs=|-+
  Is_d_ref : Outport
  Is_q_ref : Outport  Port=2
  wires:
  Sum5/1 -> Dq/1
  Sum3/1 -> Sum4/1
  Sum6/1 -> Discrete PID Controller/1
  Sum4/1 -> Discrete PID Controller3/1
  Vdc/1 -> Sum6/2
  Product/1 -> Sum4/2
  Dq/1 -> Product/1
  Qout/1 -> Sum3/2
  Activation signal/1 -> Product/2
  Vdc_ref/1 -> Sum6/1
  Discrete PID Controller3/1 -> Is_q_ref/1
  Qout_ref/1 -> Sum3/1
  Vpcc_rms_ref/1 -> Sum5/1
  Vpcc_rms/1 -> Sum5/2
  Discrete PID Controller/1 -> Is_d_ref/1

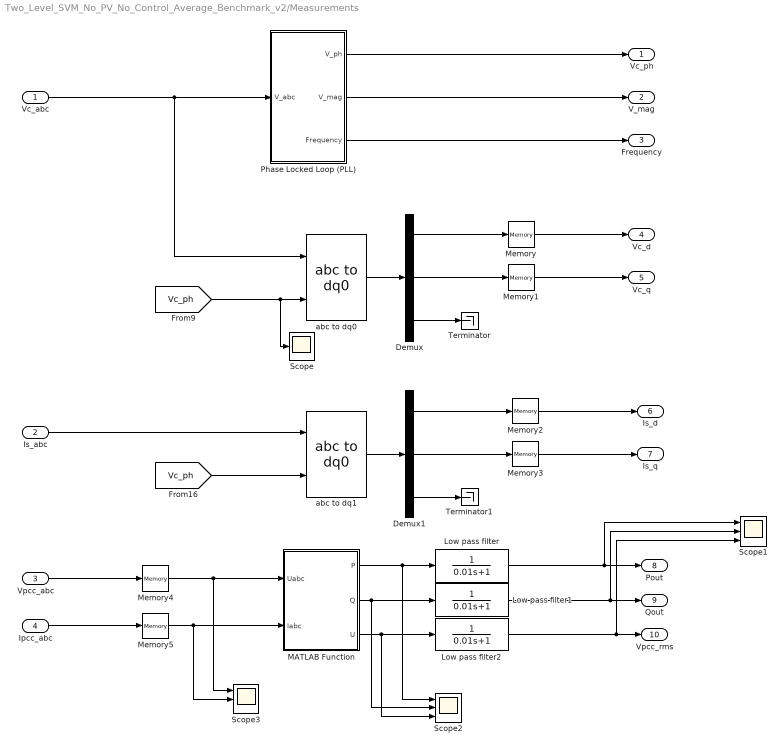
== system Two_Level_SVM_No_PV_No_Control_Average_Benchmark_v2/Measurements ==
  Vc_abc : Inport
  Is_abc : Inport  Port=2
  Vpcc_abc : Inport  Port=3
  Ipcc_abc : Inport  Port=4
  Demux : Demux  Outputs=3
  Demux1 : Demux  Outputs=3
  Low pass filter : TransferFcn  Denominator=[0.01 1]
  Low pass filter1 : TransferFcn  Denominator=[0.01 1]
  Low pass filter2 : TransferFcn  Denominator=[0.01 1]
  MATLAB Function : MATLAB Function  TreatAsAtomicUnit=on
  Memory{,1..5} (6 alike) : Memory
  Phase Locked Loop (PLL) : Subsystem
  Scope : Scope
  Scope1 : Scope  NumInputPorts=3
  Scope2 : Scope  NumInputPorts=3
  Scope3 : Scope  NumInputPorts=3
  Terminator : Terminator
  Terminator1 : Terminator
  abc to dq0 : spsabctodq0Lib/abc to dq0  Alignment=Aligned with phase A axis
  abc to dq1 : spsabctodq0Lib/abc to dq0  Alignment=Aligned with phase A axis
  Vc_ph : Outport
  V_mag : Outport  Port=2
  Frequency : Outport  Port=3
  Vc_d : Outport  Port=4
  Vc_q : Outport  Port=5
  Is_d : Outport  Port=6
  Is_q : Outport  Port=7
  Pout : Outport  Port=8
  Qout : Outport  Port=9
  Vpcc_rms : Outport  Port=10
  wires:
  Demux1/3 -> Terminator1/1
  Vc_abc/1 -> abc to dq0/1, Phase Locked Loop (PLL)/1(V_abc)
  abc to dq1/1 -> Demux1/1
  abc to dq0/1 -> Demux/1
  Demux/3 -> Terminator/1
  Phase Locked Loop (PLL)/1(V_ph) -> Vc_ph/1
  Phase Locked Loop (PLL)/3(Frequency) -> Frequency/1
  Phase Locked Loop (PLL)/2(V_mag) -> V_mag/1
  Is_abc/1 -> abc to dq1/1
  [Vc_ph] -> Scope/1, abc to dq0/2
  [Vc_ph] -> abc to dq1/2
  MATLAB Function/1(P) -> Scope2/1, Low pass filter/1
  Low pass filter/1 -> Scope1/1, Pout/1
  MATLAB Function/2(Q) -> Scope2/2, Low pass filter1/1
  Low pass filter1/1 -> Scope1/2, Qout/1
  MATLAB Function/3(U) -> Scope2/3, Low pass filter2/1
  Low pass filter2/1 -> Scope1/3, Vpcc_rms/1
  Demux/2 -> Memory1/1
  Memory1/1 -> Vc_q/1
  Demux/1 -> Memory/1
  Memory/1 -> Vc_d/1
  Demux1/1 -> Memory2/1
  Memory2/1 -> Is_d/1
  Demux1/2 -> Memory3/1
  Memory3/1 -> Is_q/1
  Vpcc_abc/1 -> Memory4/1
  Memory4/1 -> Scope3/1, MATLAB Function/1(Uabc)
  Ipcc_abc/1 -> Memory5/1
  Memory5/1 -> Scope3/2, MATLAB Function/2(Iabc)

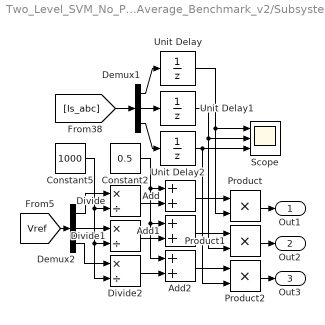
== system Two_Level_SVM_No_PV_No_Control_Average_Benchmark_v2/Subsystem ==
  Add : Sum
  Add1 : Sum
  Add2 : Sum
  Constant2 : Constant  Value=0.5  SampleTime=-1
  Constant5 : Constant  Value=1000  SampleTime=-1
  Demux1 : Demux  Outputs=3
  Demux2 : Demux  Outputs=3
  Divide : Product  Inputs=*/
  Divide1 : Product  Inputs=*/
  Divide2 : Product  Inputs=*/
  Product : Product
  Product1 : Product
  Product2 : Product
  Scope : Scope  NumInputPorts=3
  Unit Delay : UnitDelay  SampleTime=-1  HasFrameUpgradeWarning=on
  Unit Delay1 : UnitDelay  SampleTime=-1  HasFrameUpgradeWarning=on
  Unit Delay2 : UnitDelay  SampleTime=-1  HasFrameUpgradeWarning=on
  Out1 : Outport
  Out2 : Outport  Port=2
  Out3 : Outport  Port=3
  wires:
  Unit Delay/1 -> Product/2, Scope/1
  Add2/1 -> Product2/1
  Divide/1 -> Add/2
  Constant2/1 -> Add/1, Add2/1, Add1/1
  [Vref] -> Demux2/1
  Unit Delay2/1 -> Scope/3, Product2/2
  Unit Delay1/1 -> Product1/2, Scope/2
  Add1/1 -> Product1/1
  Constant5/1 -> Divide/2, Divide1/2, Divide2/2
  Demux2/1 -> Divide/1
  Demux2/2 -> Divide1/1
  Demux2/3 -> Divide2/1
  Demux1/3 -> Unit Delay2/1
  Product2/1 -> Out3/1
  Add/1 -> Product/1
  Demux1/1 -> Unit Delay/1
  [Is_abc] -> Demux1/1
  Demux1/2 -> Unit Delay1/1
  Product1/1 -> Out2/1
  Product/1 -> Out1/1
  Divide1/1 -> Add1/2
  Divide2/1 -> Add2/2

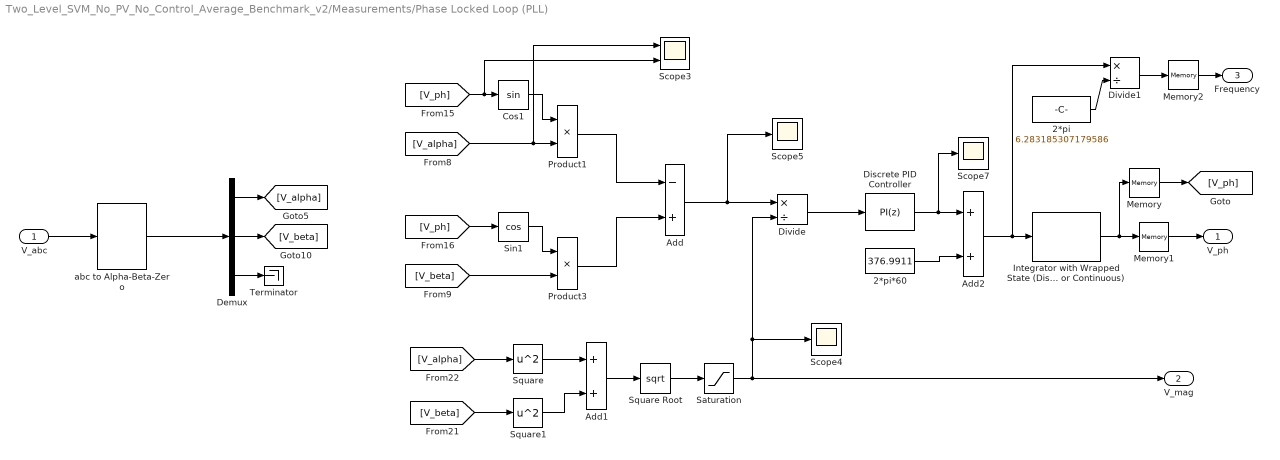
== system Two_Level_SVM_No_PV_No_Control_Average_Benchmark_v2/Measurements/Phase Locked Loop (PLL) ==
  V_abc : Inport
  2*pi : Constant  Value=6.283185307179586
  2*pi*60 : Constant  Value=376.9911
  Add : Sum  Inputs=-+
  Add1 : Sum
  Add2 : Sum
  Cos1 : Trigonometry
  Demux : Demux  Outputs=3
  Discrete PID Controller : slpidlib/PID Controller  Controller=PI  Form=Parallel  TimeDomain=Discrete-time  UseExternalTs=off  SampleTime=-1  IntegratorMethod=Forward Euler  FilterMethod=Forward Euler  ControllerParametersSource=internal  P=Kp_PLL  I=Ki_PLL  UseKiTs=off  D=0  N=100  UseFilter=on  TunerSelectOption=Transfer Function Based (PID Tuner App)  InitialConditionSource=internal  InitialConditionForIntegrator=0  InitialConditionForFilter=0  DifferentiatorICPrevScaledInput=0  ExternalReset=none  TrackingMode=off  Kt=1  LimitOutput=off  SatLimitsSource=internal  UpperSaturationLimit=inf  LowerSaturationLimit=-inf  LinearizeAsGain=off  AntiWindupMode=none  Kb=1  LimitIntegrator=off  UpperIntegratorSaturationLimit=inf  LowerIntegratorSaturationLimit=-inf  POutMin=[]  POutMax=[]  IOutMin=[]  IOutMax=[]  DOutMin=[]  DOutMax=[]  NOutMin=[]  NOutMax=[]  SumOutMin=[]  SumOutMax=[]  SaturationOutMin=[]  SaturationOutMax=[]  PParamMin=[]  PParamMax=[]  IParamMin=[]  IParamMax=[]  DParamMin=[]  DParamMax=[]  NParamMin=[]  NParamMax=[]  KbParamMin=[]  KbParamMax=[]  KtParamMin=[]  KtParamMax=[]  KbOutMin=[]  KbOutMax=[]  KtOutMin=[]  KtOutMax=[]  IntegratorOutMin=[]  IntegratorOutMax=[]  FilterOutMin=[]  FilterOutMax=[]  SumI1OutMin=[]  SumI1OutMax=[]  SumI2OutMin=[]  SumI2OutMax=[]  SumI3OutMin=[]  SumI3OutMax=[]  SumI4OutMin=[]  SumI4OutMax=[]  SumDOutMin=[]  SumDOutMax=[]  DifferentiatorOutMin=[]  DifferentiatorOutMax=[]  FilterDiffOutCoefMin=[]  FilterDiffOutCoefMax=[]  ReciprocalOutMin=[]  ReciprocalOutMax=[]  SumDenOutMin=[]  SumDenOutMax=[]  SumNumOutMin=[]  SumNumOutMax=[]  DivideOutMin=[]  DivideOutMax=[]  UdiffTsProdOutMin=[]  UdiffTsProdOutMax=[]  NTsProdOutMin=[]  NTsProdOutMax=[]  UintegralTsProdOutMin=[]  UintegralTsProdOutMax=[]  UngainTsProdOutMin=[]  UngainTsProdOutMax=[]  ClampingZeroOutDataTypeStr=Inherit: Inherit via back propagation  ClampingZeroOutMin=[]  ClampingZeroOutMax=[]  FilterDenConstantOutDataTypeStr=Inherit: Inherit via back propagation  FilterDenConstantOutMin=[]  FilterDenConstantOutMax=[]  PCopyOutDataTypeStr=Inherit: Inherit via back propagation  PCopyOutMin=[]  PCopyOutMax=[]  NCopyOutDataTypeStr=Inherit: Inherit via back propagation  NCopyOutMin=[]  NCopyOutMax=[]  IntegratorContinuousStateAttributes=''  IntegratorStateMustResolveToSignalObject=off  IntegratorRTWStateStorageClass=Auto  FilterContinuousStateAttributes=''  FilterStateMustResolveToSignalObject=off  FilterRTWStateStorageClass=Auto  ParallelPVariant=InternalParameters  IdealPVariant=Disabled  IVariant=InternalParameters  DVariant=Disabled  IntegratorVariant=Discrete  SatVariant=Disabled  AWVariant=Passthrough  PCopyVariant=Disabled  TRVariant=Disabled  FdbkBlocksVariant=Forward  IdealPFdbkVariant=Disabled  SatFdbkVariant=Disabled  DerivativeFilterVariant=Disabled  NVariant=Disabled  NCopyVariant=Disabled_SignalSpec  FilterICVariant=Disabled  IntegratorICVariant=InternalICs  ExternalResetVariant=Disabled  TRSumVariant=Passthrough  SumFdbkVariant=Disabled  SumVariant=Sum_PI  TsampFilterVariant=InternalTs  TsampNgainVariant=Passthrough  TsampIntegralVariant=Passthrough  ExternalSaturationOutDataTypeStr=Inherit: Same as second input
  Divide : Product  Inputs=*/
  Divide1 : Product  Inputs=*/
  Integrator with Wrapped State (Discrete or Continuous) : eeGeneralControl/Integrator with Wrapped State (Discrete or Continuous)  LabelModeActiveChoice=Discrete  WrappedStateUpperValue=pi  WrappedStateLowerValue=-pi  x0=0  Ts=-1
  Memory : Memory
  Memory1 : Memory
  Memory2 : Memory
  Product1 : Product
  Product3 : Product
  Saturation : Saturate  UpperLimit=1e10  LowerLimit=0.001
  Scope3 : Scope  NumInputPorts=2
  Scope4 : Scope
  Scope5 : Scope
  Scope7 : Scope
  Sin1 : Trigonometry  Operator=cos
  Square : Math  Operator=square
  Square Root : Sqrt
  Square1 : Math  Operator=square
  Terminator : Terminator
  abc to Alpha-Beta-Zero : spsabctoAlphaBetaZeroLib/abc to Alpha-Beta-Zero
  V_ph : Outport
  V_mag : Outport  Port=2
  Frequency : Outport  Port=3
  wires:
  Saturation/1 -> V_mag/1, Scope4/1, Divide/2
  [V_alpha] -> Square/1
  Discrete PID Controller/1 -> Scope7/1, Add2/1
  Cos1/1 -> Product1/1
  abc to Alpha-Beta-Zero/1 -> Demux/1
  Demux/1 -> [V_alpha]
  [V_alpha] -> Scope3/1, Product1/2
  Square/1 -> Add1/1
  Demux/2 -> [V_beta]
  V_abc/1 -> abc to Alpha-Beta-Zero/1
  Product3/1 -> Add/2
  [V_ph] -> Scope3/2, Cos1/1
  [V_beta] -> Product3/2
  Add2/1 -> Divide1/1, Integrator with Wrapped State (Discrete or Continuous)/1
  Square1/1 -> Add1/2
  [V_ph] -> Sin1/1
  Demux/3 -> Terminator/1
  Product1/1 -> Add/1
  Add/1 -> Scope5/1, Divide/1
  Sin1/1 -> Product3/1
  2*pi*60/1 -> Add2/2
  Add1/1 -> Square Root/1
  Square Root/1 -> Saturation/1
  [V_beta] -> Square1/1
  Divide/1 -> Discrete PID Controller/1
  Integrator with Wrapped State (Discrete or Continuous)/1 -> Memory1/1, Memory/1
  2*pi/1 -> Divide1/2
  Memory/1 -> [V_ph]
  Memory1/1 -> V_ph/1
  Memory2/1 -> Frequency/1
  Divide1/1 -> Memory2/1

== matlab function Two_Level_SVM_No_PV_No_Control_Average_Benchmark_v2/Measurements/MATLAB Function ==
  data: Uabc input; P output; Iabc input; Q output; U output
function [P,Q,U] = fcn(Uabc,Iabc)

Ua = Uabc(1);
Ub = Uabc(2);
Uc = Uabc(3);

Ia = Iabc(1);
Ib = Iabc(2);
Ic = Iabc(3);

P = Ua*Ia + Ub*Ib + Uc*Ic;
Q = 1/sqrt(3)*((Ua-Ub)*Ic + (Ub-Uc)*Ia + (Uc-Ua)*Ib);
U = sqrt(2)*sqrt(-Ua*Ub-Ub*Uc-Uc*Ua);
